simulink model "shoot3"  (R2017b)
settings: Solver=VariableStepAuto  StartTime=0.0  StopTime=10.0  RelTol=1e-3
settings Model: Creator=ghleila  LastModifiedBy=ghleila

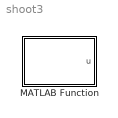
== system shoot3 ==
  MATLAB Function : MATLAB Function  TreatAsAtomicUnit=on

== matlab function shoot3/MATLAB Function ==
  data: u output
function u = fcn2

global y;
y=y+1;
u=y;
